simulink model "orbit_propagation"  (R2022b)
settings: Solver=VariableStepAuto  StartTime=0.0  StopTime=5000  RelTol=1e-13  AbsTol=1e-14
undefined symbols (not defined in the file or in its folder): environment, r0, sat, settings, v0
libraries: matrix_library x1
settings Model: Creator=brent  LastModifiedBy=brent

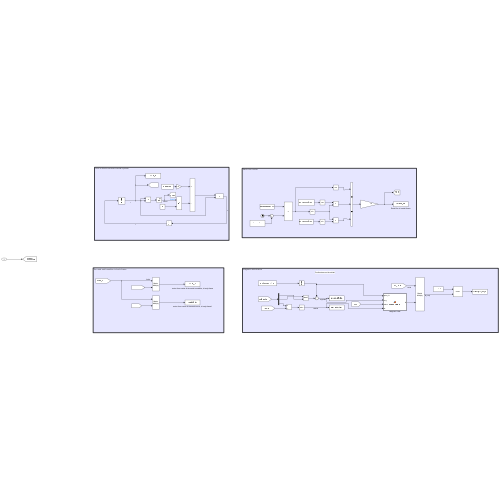
[thumbnail: Simulink's stored preview of the top-level diagram]
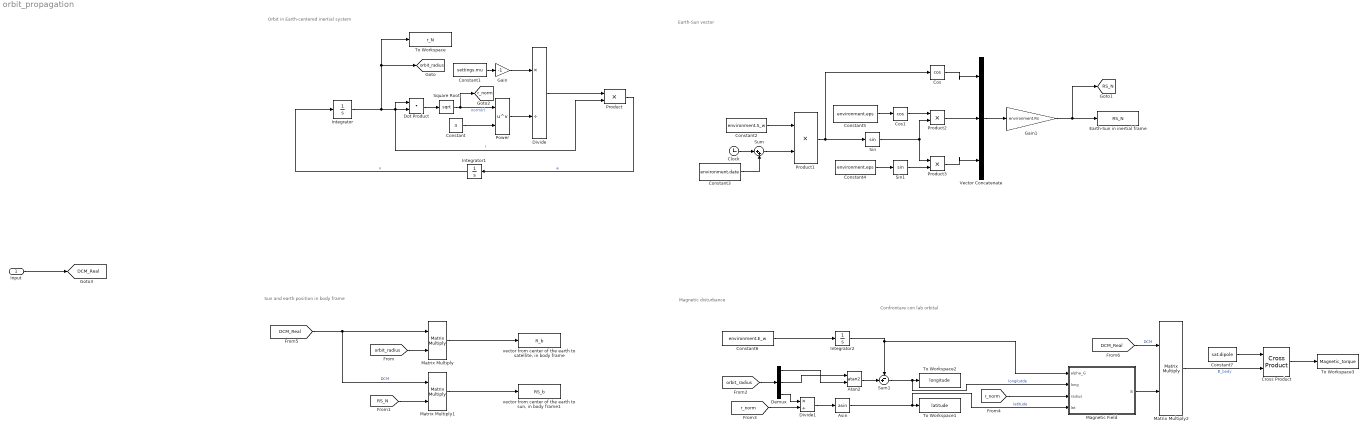
== system orbit_propagation ==
  note: Confrontare con lab orbital
  note: Magnetic disturbance
  note: Sun and earth position in body frame
  note: Earth-Sun vector
  note: Orbit in Earth-centered inertial system
  Input : Inport
  Asin : Trigonometry  Operator=asin
  Atan2 : Trigonometry  Operator=atan2
  Clock : Clock
  Constant : Constant  Value=3
  Constant1 : Constant  Value=settings.mu
  Constant2 : Constant  Value=environment.S_w
  Constant3 : Constant  Value=environment.date
  Constant4 : Constant  Value=environment.eps
  Constant5 : Constant  Value=environment.eps
  Constant6 : Constant  Value=environment.E_w
  Constant7 : Constant  Value=sat.dipole
  Cos : Trigonometry  Operator=cos
  Cos1 : Trigonometry  Operator=cos
  Cross Product : matrix_library/Cross Product
  Demux : Demux  Outputs=3
  Divide : Product  Inputs=*/
  Divide1 : Product  Inputs=*/
  Dot Product : DotProduct  OutDataTypeStr=Inherit: Inherit via internal rule
  Earth-Sun in inertial frame : ToWorkspace  VariableName=RS_N  SaveFormat=Timeseries  SampleTime=-1
  Gain : Gain  Gain=-1
  Gain1 : Gain  Gain=environment.Rs
  Integrator : Integrator  InitialCondition=r0
  Integrator1 : Integrator  InitialCondition=v0
  Integrator2 : Integrator  InitialCondition=environment.theta_G0
  Magnetic Field : MATLAB Function  TreatAsAtomicUnit=on
  Matrix Multiply : Product  Multiplication=Matrix(*)
  Matrix Multiply1 : Product  Multiplication=Matrix(*)
  Matrix Multiply2 : Product  Multiplication=Matrix(*)
  Power : Math  Operator=pow
  Product{,1..3} (4 alike) : Product
  Sin : Trigonometry
  Sin1 : Trigonometry
  Square Root : Sqrt
  Sum : Sum  Inputs=|++
  Sum1 : Sum  Inputs=-+|
  To Workspace : ToWorkspace  VariableName=r_N  SampleTime=-1
  To Workspace1 : ToWorkspace  VariableName=latitude  SampleTime=-1
  To Workspace2 : ToWorkspace  VariableName=longitude  SampleTime=-1
  To Workspace3 : ToWorkspace  VariableName=Magnetic_torque  SaveFormat=Timeseries  SampleTime=-1
  Vector Concatenate : Concatenate  NumInputs=3
  "vector from center of the earth to satellite, in body frame" : ToWorkspace  VariableName=R_b  SampleTime=-1
  "vector from center of the earth to sun, in body frame1" : ToWorkspace  VariableName=RS_b  SampleTime=-1
  tag scope: DCM_Real=global, RS_N=global, orbit_radius=global, r_norm=global
  wires:
  Integrator/1 -> [orbit_radius], To Workspace/1, Product/2, Dot Product/2, Dot Product/1  "r"
  Integrator1/1 -> Integrator/1  "v"
  Dot Product/1 -> Square Root/1
  Square Root/1 -> [r_norm], Power/1  "norm(r)"
  Constant1/1 -> Gain/1
  Gain/1 -> Divide/1
  Power/1 -> Divide/2
  Divide/1 -> Product/1
  Product/1 -> Integrator1/1  "a"
  Constant/1 -> Power/2
  [DCM_Real] -> Matrix Multiply/1, Matrix Multiply1/1  "DCM"
  Matrix Multiply/1 -> "vector from center of the earth to satellite, in body frame"/1
  Constant2/1 -> Product1/1
  Clock/1 -> Sum/1
  Constant3/1 -> Sum/2
  Sum/1 -> Product1/2
  Product1/1 -> Sin/1, Cos/1
  Constant5/1 -> Cos1/1
  Constant4/1 -> Sin1/1
  Sin1/1 -> Product3/2
  Cos1/1 -> Product2/1
  Sin/1 -> Product3/1, Product2/2
  Product3/1 -> Vector Concatenate/3
  Product2/1 -> Vector Concatenate/2
  Cos/1 -> Vector Concatenate/1
  Vector Concatenate/1 -> Gain1/1
  Gain1/1 -> [RS_N], Earth-Sun in inertial frame/1
  [orbit_radius] -> Matrix Multiply/2
  Matrix Multiply1/1 -> "vector from center of the earth to sun, in body frame1"/1
  [RS_N] -> Matrix Multiply1/2
  [orbit_radius] -> Demux/1
  Demux/3 -> Divide1/1
  [r_norm] -> Divide1/2
  Divide1/1 -> Asin/1
  Asin/1 -> Magnetic Field/4(lat), To Workspace1/1  "latitude"
  Demux/2 -> Atan2/1
  Demux/1 -> Atan2/2
  Atan2/1 -> Sum1/2
  Integrator2/1 -> Sum1/1, Magnetic Field/1(alpha_G)
  Constant6/1 -> Integrator2/1
  Sum1/1 -> Magnetic Field/2(long), To Workspace2/1  "longitutde"
  [r_norm] -> Magnetic Field/3(radius)
  Input/1 -> [DCM_Real]
  [DCM_Real] -> Matrix Multiply2/1  "DCM"
  Magnetic Field/1(B) -> Matrix Multiply2/2
  Matrix Multiply2/1 -> Cross Product/2  "B_body"
  Constant7/1 -> Cross Product/1
  Cross Product/1 -> To Workspace3/1

== matlab function orbit_propagation/Magnetic Field ==
  data: alpha_G input; long input; radius input; B output; lat input; environment parameter; settings parameter
function B = magneticField(alpha_G,long,radius,lat,environment,settings)
%{  
    Return the magnetic field component in inertial reference frame

%}
theta = (pi/2-lat);     % theta is the colatitude [rad]
alpha = long + alpha_G; 

g = environment.WMM.g;
h = environment.WMM.h;
K = environment.WMM.K;
R = environment.R;
N = settings.N;

%% P-dP
% validated through the P and dP tables in "Jeremy Davis, Mathematical Modeling of Earthas Magnetic
% Field, 2004"

%%%%%%%%%%%%%%%%%%%%%%%%%%%%%%%%%%%%%%%%%%%%%%%%%%%%%%%%%%%%%%%%%%%%%%%%%%%%%%%%%%%%%%%%%%%%%%%%
% P_{(n),(m+1)}: 
% given P(a,b) -> n=a, m=b-1
% n from 1 to N
% m from 0 to N
% N order of accuracy
%%%%%%%%%%%%%%%%%%%%%%%%%%%%%%%%%%%%%%%%%%%%%%%%%%%%%%%%%%%%%%%%%%%%%%%%%%%%%%%%%%%%%%%%%%%%%%%%

P = zeros(N,N+1);
dP = zeros(N,N+1);

P_00 = 1;
dP_00 = 0;

P_01 = 0; 
dP_01 = 0;

P(1,1) = cos(theta); % n=1, m=0
dP(1,1) = -sin(theta)*P_00; 

P(1,2) = sin(theta);  % n=1, m=1
dP(1,2) = cos(theta)*P_00;

for i = 2:N % ciclo in n a partire da n=2 a n=N
    for j = 0:i % ciclo in m da m=0 a m=n
        if j == i
        P(i,j+1) = sin(theta)*P(i-1,j);
        dP(i,j+1) = sin(theta)*dP(i-1,j) + cos(theta)*P(i-1,j);
        elseif i < 3
            if j == 0 % n=2, m=0
            P(i,j+1) = cos(theta)*P(i-1,j+1) - K(i,j+1)*P_00;
            dP(i,j+1) = -sin(theta)*P(i-1,j+1) + cos(theta)*dP(i-1,j+1) ...
                - K(i,j+1)*dP_00;
            elseif j == 1 % n=2, m=1
                P(i,j+1) = cos(theta)*P(i-1,j+1) - K(i,j+1)*P_01;
                dP(i,j+1) = -sin(theta)*P(i-1,j+1) + cos(theta)*dP(i-1,j+1)...
                    - K(i,j+1)*dP_01;
            end
        else
            P(i,j+1) = cos(theta)*P(i-1,j+1) - K(i,j+1)*P(i-2,j+1);
            dP(i,j+1) = -sin(theta)*P(i-1,j+1) + cos(theta)*dP(i-1,j+1) ...
                - K(i,j+1)*dP(i-2,j+1);
        end
    end
end

%% Magnetic Field

B_r = 0;
B_th = 0;
B_phi = 0;

%indice i scorre n da 1 a N
%indice j scorre m da 0 a n

for m = 0:N
    for n = 1:N
        if m<=n
            B_r = B_r + (R/radius)^(n+2)*(n+1)*...
                ((g(n,m+1)*cos(m*long) + h(n,m+1)*sin(m*long))*P(n, m+1));
            B_th = B_th + (R/radius)^(n+2)*...
                ((g(n,m+1)*cos(m*long) + h(n,m+1)*sin(m*long))*dP(n, m+1));
            B_phi = B_phi + (R/radius)^(n+2)*...
                (m*(-g(n,m+1)*sin(m*long) + h(n,m+1)*cos(m*long))* P(n, m+1));

        end

    end
end

B_th = -B_th;
B_phi = -B_phi/sin(theta);

B_x = ( B_r*cos(lat) + B_th*sin(lat) ) * cos(alpha) - B_phi*sin(alpha);
B_y = ( B_r*cos(lat) + B_th*sin(lat) ) * sin(alpha) + B_phi*cos(alpha);
B_z = B_r*sin(lat) + B_th*cos(lat);

B = norm([B_x B_y B_z]);
